simulink model "chalgyafzintegrationkrrhe"  (R2024b)
settings: Solver=ode4  StartTime=0.0  StopTime=150  FixedStep=0.001  RelTol=1e-3
values from neighbouring files (symbols this model uses):
  kappa = (dx .* d2y - dy .* d2x) ./          ((dx.^2 + dy.^2).^(3/2) + 1e-6)    [Buildmadrasspeedway.m]
  pathX = ppval(ppx,s)    [Buildmadrasspeedway.m]
  pathY = ppval(ppy,s)    [Buildmadrasspeedway.m]
  pathYaw = unwrap(atan2(dy,dx))    [Buildmadrasspeedway.m]
  s = 0:ds:t(end)    [Buildmadrasspeedway.m]
undefined symbols (not defined in the file or in its folder): v_ref
libraries: autolibsharedcoupling x1, vehdynlibsteering x1, autolibmappedmotor x1, vehdynlibdriver x1, autolibshared x1
(part 1 of 2)
settings Model: Creator=ASUS  LastModifiedBy=ASUS
settings DataIOCC: ReturnWorkspaceOutputs=off

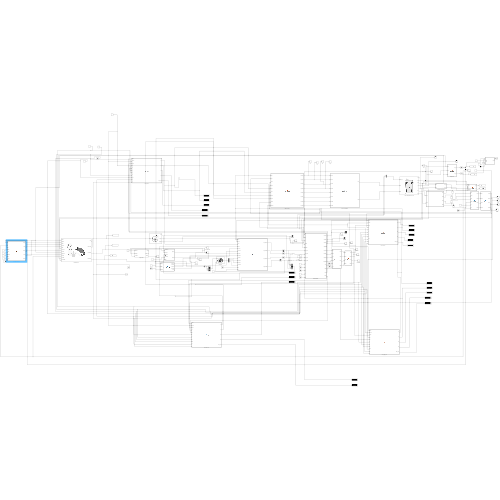
[thumbnail: Simulink's stored preview of the top-level diagram]
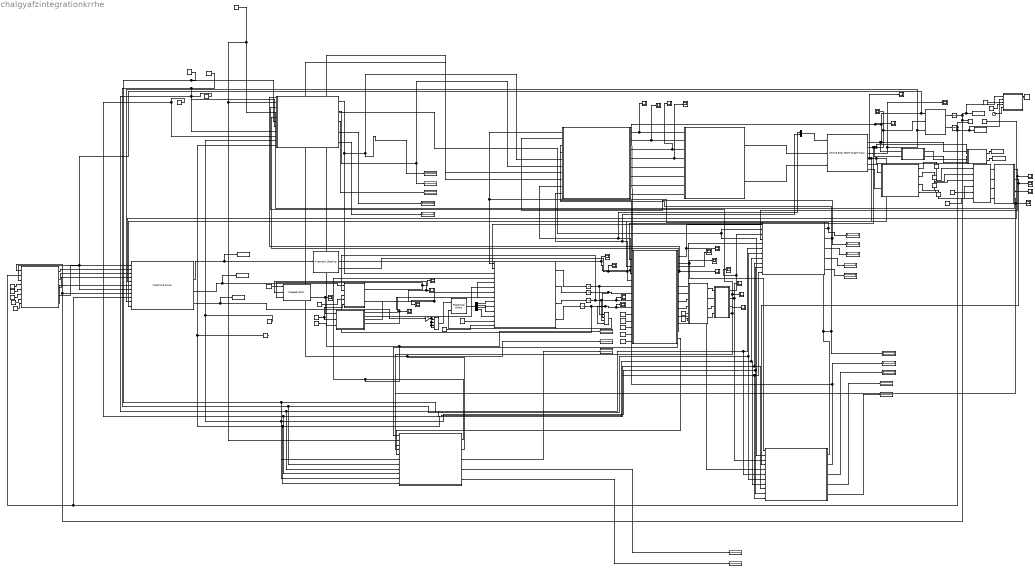
== system chalgyafzintegrationkrrhe ==
  Alpha RR : Scope
  Alpha Rl : Scope
  Bodytoworld : MATLAB Function  TreatAsAtomicUnit=on
  Clock : Clock
  Constant : Constant  Value=pathX(1)
  Constant1 : Constant  Value=0.10
  Constant10 : Constant  Value=0.001
  Constant11 : Constant  Value=0.08
  Constant12 : Constant  Value=0.03
  Constant13 : Constant  Value=0.001
  Constant14 : Constant  Value=kappa
  Constant15 : Constant  Value=pathX
  Constant16 : Constant  Value=0.3
  Constant17 : Constant  Value=0
  Constant18 : Constant  Value=pathY
  Constant19 : Constant  Value=pathYaw
  Constant2 : Constant  Value=0.08
  Constant20 : Constant  Value=v_ref
  Constant21 : Constant  Value=60
  Constant22 : Constant  Value=6
  Constant23 : Constant  Value=0.95
  Constant24 : Constant
  Constant25 : Constant  Value=pathY(1)
  Constant3 : Constant  Value=0.30
  Constant31 : Constant  Value=0.8
  Constant32 : Constant  Value=0.8
  Constant33 : Constant  Value=1.2
  Constant34 : Constant  Value=1.2
  Constant35 : Constant  Value=0.3
  Constant4 : Constant
  Constant5 : Constant  Value=1e7
  Constant6 : Constant  Value=200
  Constant7 : Constant  Value=0
  Constant9 : Constant
  Demux : Demux
  Disc Brake : autolibsharedcoupling/Rotational Brake  BrakeType=Disc  rotType=No inertia  extInfo=off  Iyy=1  br=1e-3  omegao=0  mu_static=0.4  mu_kinetic=0.35  disk_abore=0.02  Rm=0.08  num_pads=2  drum_abore=0.0508  drum_a=0.123  drum_c=0.212  drum_r=0.15  drum_theta1=0  drum_theta2=126  brake_p_bpt=[1 11.4736842105263 21.9473684210526 32.4210526315789 42.8947368421053 53.3684210526316 63.8421052631579 74.3157894736842 84.7894736842105 95.2631578947368 105.736842105263 116.210526315789 126.684210526316 137.157894736842 147.631578947368 158.105263157895 168.578947368421 179.052631578947 189.526315789474 200]  brake_n_bpt=[0 52.6315789473684 105.263157894737 157.894736842105 210.526315789474 263.157894736842 315.789473684211 368.421052631579 421.052631578947 473.684210526316 526.315789473684 578.947368421053 631.578947368421 684.210526315789 736.842105263158 789.473684210526 842.105263157895 894.736842105263 947.368421052632 1000]  f_brake_t=[43.4900602404453 42.5056030554862 41.5350898940194 40.5780454442085 39.6340111501808 38.7025443887544 37.7832176914519 36.8756180088306 35.9793460143796 35.0940154454303 34.2192524787115 33.3546951383474 32.4999927342521 31.6548053290159 30.8188032315107 29.991666515561 29.1730845621415 28.362755623661 27.5603864089927 26.765691687993;498.991217495636 487.695866636631 476.560505099801 465.579679307235 454.748127933653 444.060772460445 433.51270824929 423.099196101319 412.81565427025 402.657650900201 392.620896861006 382.701238955775 372.894653477208 363.197240090814 353.605216024701 344.114910546964 334.722759712992 325.425301366216 316.219170376863 307.10109410434;954.492374750826 932.886130217776 911.585920305583 890.581313170261 869.862244717126 849.419000532136 829.242198807128 809.322774193808 789.651962526121 770.221286354971 751.0225412433 732.047782773203 713.289314220164 694.739674852612 676.391628817892 658.238154578366 640.272434863842 622.48784710877 604.877954344734 587.436496520688;1409.99353200602 1378.07639379892 1346.61133551136 1315.58294703329 1284.9763615006 1254.77722860383 1224.97168936497 1195.5463522863 1166.48827078199 1137.78492180974 1109.42418562559 1081.39432659063 1053.68397496312 1026.28210961441 999.178041611083 972.361398609768 945.822110014692 919.550392851325 893.536738312604 867.771898937035;1865.49468926121 1823.26665738007 1781.63675071715 1740.58458089631 1700.09047828407 1660.13545667552 1620.7011799228 1581.76993037878 1543.32457903786 1505.34855726451 1467.82583000789 1430.74087040806 1394.07863570608 1357.82454437621 1321.96445440427 1286.48464264117 1251.37178516554 1216.61293859388 1182.19552228048 1148.10730135338;2320.9958465164 2268.45692096121 2216.66216592293 2165.58621475934 2115.20459506754 2065.49368474721 2016.43067048064 1967.99350847127 1920.16088729373 1872.91219271928 1826.22747439018 1780.08741422549 1734.47329644903 1689.36697913801 1644.75086719747 1600.60788667257 1556.92146031639 1513.67548433643 1470.85430624835 1428.44270376973;2776.49700377159 2713.64718454235 2651.68758112871 2590.58784862237 2530.31871185102 2470.8519128189 2412.16016103848 2354.21708656376 2296.9971955496 2240.47582817405 2184.62911877248 2129.43395804292 2074.86795719199 2020.9094138998 1967.53727999066 1914.73113070398 1862.47113546724 1810.73803007899 1759.51309021622 1708.77810618608;3231.99816102678 3158.8374481235 3086.71299633449 3015.58948248539 2945.43282863449 2876.21014089059 2807.88965159632 2740.44066465625 2673.83350380547 2608.03946362882 2543.03076315477 2478.78050186034 2415.26261793494 2352.4518486616 2290.32369278385 2228.85437473538 2168.02081061809 2107.80057582154 2048.17187418409 1989.11350860242;3687.49931828197 3604.02771170464 3521.73841154027 3440.59111634842 3360.54694541796 3281.56836896228 3203.61914215416 3126.66424274874 3050.66981206134 2975.60309908359 2901.43240753707 2828.12704567777 2755.6572786779 2683.9942834234 2613.11010557704 2542.97761876678 2473.57048576894 2404.8631215641 2336.83065815196 2269.44891101877;4143.00047553716 4049.21797528579 3956.76382674606 3865.59275021144 3775.66106220143 3686.92659703397 3599.34863271199 3512.88782084123 3427.50612031721 3343.16673453836 3259.83405191936 3177.4735894952 3096.05193942085 3015.5367181852 2935.89651837023 2857.10086279818 2779.12016091979 2701.92566730665 2625.48944211983 2549.78431343512;4598.50163279235 4494.40823886693 4391.78924195184 4290.59438407447 4190.77517898491 4092.28482510566 3995.07812326983 3899.11139893372 3804.34242857308 3710.73036999313 3618.23569630166 3526.82013331263 3436.44660016381 3347.079152947 3258.68293116342 3171.22410682959 3084.66983607064 2998.98821304921 2914.1482260877 2830.11971585147;5054.00279004754 4939.59850244808 4826.81465715762 4715.59601793749 4605.88929576838 4497.64305317735 4390.80761382767 4285.3349770262 4181.17873682896 4078.2940054479 3976.63734068395 3876.16667713006 3776.84126090677 3678.62158770879 3581.46934395661 3485.34735086099 ...(+2764 chars)]  aMode=2
      settings: LibrarySourceBlock=vehdynlibbrake/Disc Brake
  Display{,1..19} (20 alike) : Display
  FZFL : Scope
  FZFR : Scope
  FZRL : Scope
  FZRR : Scope
  "Force FWF and FWR " : MATLAB Function  TreatAsAtomicUnit=on
  Front_Left_tire : MATLAB Function  TreatAsAtomicUnit=on
  Front_Right_Tire : MATLAB Function  TreatAsAtomicUnit=on
  Gain : Gain  Gain=8e+6
  Integrator{,1..2,4} (4 alike) : Integrator  InitialCondition=0.1/0.3
  Integrator3 : Integrator  InitialCondition=pathX(1)
  Integrator5 : Integrator  InitialCondition=pathY(1)
  KAPPA FL : Scope
  KAPPA FR : Scope
  KAPPA RL : Scope
  KAPPA RR : Scope
  Kinematic Steering : vehdynlibsteering/Kinematic Steering  StrgType=Ackerman  StrgRatioType=Constant  Loc=Front  NrmlFctr=0.01  TrckWdth=1.2  WhlBase=1.6  Db=0  StrgRng=deg2rad(25)  StrgAngBpts="[-6.2832   -5.0265   -3.7699   -2.5133   -1.2566         0    1.2566    2.5133    3.7699    5.0265    6.2832]"  StrgRatioTbl=|  StrgRatio=1  PctAckIn=off  PctAck=100  PctAckTbl=ones(1,11)*100  StrgArmLngth=0.1  RckCsLngth=0.5  TieRodLngth=0.248  D=0.2  PnnRadius=0.00085818  PnnRadiusTbl="[0.0055    0.0055    0.0056    0.0057    0.0058    0.0057    0.0057    0.0057    0.0056    0.0055    0.0055]"  RodLngth=0.1  ParaArmLngth=0.9  aMode=2
      | [13.5000   13.3750   13.2500   13.1250   13.0000   13.0000   13.0000   13.1250   13.2500   13.3750   13.5000
      | ]
  MATLAB Function : MATLAB Function  TreatAsAtomicUnit=on
  MATLAB Function1 : MATLAB Function  TreatAsAtomicUnit=on
  MATLAB Function10 : MATLAB Function  TreatAsAtomicUnit=on
  MATLAB Function2 : MATLAB Function  TreatAsAtomicUnit=on
  MATLAB Function3 : MATLAB Function  TreatAsAtomicUnit=on  SystemSampleTime=0.001
  MATLAB Function4 : MATLAB Function  TreatAsAtomicUnit=on
  MATLAB Function5 : MATLAB Function  TreatAsAtomicUnit=on  SystemSampleTime=0.001
  MATLAB Function6 : MATLAB Function  TreatAsAtomicUnit=on
  MATLAB Function7 : MATLAB Function  TreatAsAtomicUnit=on
  MATLAB Function8 : MATLAB Function  TreatAsAtomicUnit=on
  MATLAB Function9 : MATLAB Function  TreatAsAtomicUnit=on
  Mapped Motor : autolibmappedmotor/Mapped Motor  w_Tmax_bp_ext=w_Tmax_bp  Tmax_w_V_ext=Tmax_w_V  w_Tmin_bp_ext=w_Tmin_bp  Tmin_w_V_ext=Tmin_w_V  port_config=Speed  param_by=Maximum torque and power  w_t=[ 0 375 750 800 ]  T_t=[0.09 0.08 0.07 0]  torque_max=60  power_max=35000  SpreadsheetTqLimitsFileName=MotorCalibrationImportData.xlsx  Tmax_w_V=[0.09 0.09 0.09;0.08 0.08 0.08;0.07 0.07 0.07;0 0 0]  w_Tmax_bp=[ 0 375 750 800 ]  V_Tmax_bp=[500 750 900]  Tmin_w_V=[-0.09 -0.09 -0.09;-0.08 -0.08 -0.08;-0.07 -0.07 -0.07;0 0 0]  w_Tmin_bp=[ 0 375 750 800 ]  V_Tmin_bp=[500 750 900]  Tc=0.02  param_loss=Single efficiency measurement  SpreadsheetLossFileName=MotorCalibrationImportData.xlsx  SpreadsheetEffFileName=MotorCalibrationImportData.xlsx  eff=100  w_eff=375  T_eff=0.08  Piron=0  Pbase=0  w_eff_bp=[-8000 -4000 0 4000 8000]  T_eff_bp=[0 0.03 0.06 0.09]  Temp_eff_bp=[233.15 293.15 373.15]  V_eff_bp=[500 700 900]  losses_table=[1.49 1.67 2.21 3.10; 0.42 0.69 1.14 2.03; 0.06 0.24 0.78 1.68; 0.42 0.69 1.14 2.03; 1.49 1.67 2.21 3.10]  losses_table_3d=cat(3,1.05*[1.49 1.67 2.21 3.10; 0.42 0.69 1.14 2.03; 0.06 0.24 0.78 1.68; 0.42 0.69 1.14 2.03; 1.49 1.67 2.21 3.10],[1.49 1.67 2.21 3.10; 0.42 0.69 1.14 2.03; 0.06 0.24 0.78 1.68; 0.42 0.69 1.14 2.03; 1.49 1.67 2.21 3.10],1.03*[1.49 1.67 2.21 3.10; 0.42 0.69 1.14 2.03; 0.06 0.24 0.78 1.68; 0.42 0.69 1.14 2.03; 1.49 1.67 2.21 3.10])  losses_table_4d=cat(4,cat(3,[1.5645 0.441 0.063 0.441 1.5645;1.7535 0.7245 0.252 0.7245 1.7535;2.3205 1.197 0.819 1.197 2.3205;3.255 2.1315 1.764 2.1315 3.255],[1.5645 0.441 0.063 0.441 1.5645;1.7535 0.7245 0.252 0.7245 1.7535;2.3205 1.197 0.819 1.197 2.3205;3.255 2.1315 1.764 2.1315 3.255],[1.5645 0.441 0.063 0.441 1.5645;1.7535 0.7245 0.252 0.7245 1.7535;2.3205 1.197 0.819 1.197 2.3205;3.255 2.1315 1.764 2.1315 3.255]),cat(3,[1.49 0.42 0.06 0.42 1.49;1.67 0.69 0.24 0.69 1.67;2.21 1.14 0.78 1.14 2.21;3.1 2.03 1.68 2.03 3.1],[1.49 0.42 0.06 0.42 1.49;1.67 0.69 0.24 0.69 1.67;2.21 1.14 0.78 1.14 2.21;3.1 2.03 1.68 2.03 3.1],[1.49 0.42 0.06 0.42 1.49;1.67 0.69 0.24 0.69 1.67;2.21 1.14 0.78 1.14 2.21;3.1 2.03 1.68 2.03 3.1]),cat(3,[1.5347 0.4326 0.0618 0.4326 1.5347;1.7201 0.7107 0.2472 0.7107 1.7201;2.2763 1.1742 0.8034 1.1742 2.2763;3.193 2.0909 1.7304 2.0909 3.193],[1.5347 0.4326 0.0618 0.4326 1.5347;1.7201 0.7107 0.2472 0.7107 1.7201;2.2763 1.1742 0.8034 1.1742 2.2763;3.193 2.0909 1.7304 2.0909 3.193],[1.5347 0.4326 0.0618 0.4326 1.5347;1.7201 0.7107 0.2472 0.7107 1.7201;2.2763 1.1742 0.8034 1.1742 2.2763;3.193 2.0909 1.7304 2.0909 3.193]))  efficiency_table=[95 95 95 95; 95 95 95 95; 95 95 95 95; 95 95 95 95; 95 95 95 95]  efficiency_table_3d=cat(3,90*ones(5,4),95*ones(5,4),92*ones(5,4))  efficiency_table_4d=cat(4,cat(3,90*ones(5,4)',90*ones(5,4)',90*ones(5,4)'),cat(3,95*ones(5,4)',95*ones(5,4)',95*ones(5,4)'),cat(3,92*ones(5,4)',92*ones(5,4)',92*ones(5,4)'))  J=5e-6  b=1e-5  omega_o=0  T_t_extended=[0 0.07 0.08 0.09 0.08 0.07 0]  w_t_extended=[-800 -750 -375 0 375 750 800]  KLossIron=0  KLossCopper=0  x_w_eff_vec=[-8000 -4000 0 4000 8000]  x_T_eff_vec=[-0.09 -0.06 -0.03 0 0.03 0.06 0.09]  x_tmp_eff_vec=[233.15 293.15 373.15]  x_V_eff_vec=[500 700 900]  x_losses_mat=[3.1 2.21 1.67 1.49 1.67 2.21 3.1;2.03 1.14 0.69 0.42 0.69 1.14 2.03;1.68 0.78 0.24 0.06 0.24 0.78 1.68;2.03 1.14 0.69 0.42 0.69 1.14 2.03;3.1 2.21 1.67 1.49 1.67 2.21 3.1]  x_losses_mat_3d=cat(3,[3.255 2.3205 1.7535 1.5645 1.7535 2.3205 3.255;2.1315 1.197 0.7245 0.441 0.7245 1.197 2.1315;1.764 0.819 0.252 0.063 0.252 0.819 1.764;2.1315 1.197 0.7245 0.441 0.7245 1.197 2.1315;3.255 2.3205 1.7535 1.5645 1.7535 2.3205 3.255],[3.1 2.21 1.67 1.49 1.67 2.21 3.1;2.03 1.14 0.69 0.42 0.69 1.14 2.03;1.68 0.78 0.24 0.06 0.24 0.78 1.68;2.03 1.14 0.69 0.42 0.69 1.14 2.03;3.1 2.21 1.67 1.49 1.67 2.21 3.1],[3.193 2.2763 1.7201 1.5347 1.7201 2.2763 3.193;2.0909 1.1742 0.7107 0.4326 0.7107 1.1742 2.0909;1.7304 0.8034 0.2472 0.0618 0.2472 0.8034 1.7304;2.0909 1.1742 0.7107 0.4326 0.7107 1.1742 2.0909;3.193 2.2763 1.7201 1.5347 1.7201 2.2763 3.193])  x_losses_mat_4d=cat(4,cat(3,[1.5645 0.441 0.063 0.441 1.5645;1.7535 0.7245 0.252 0.7245 1.7535;2.3205 1.197 0.819 1.197 2.3205;3.255 2.1315 1.764 2.1315 3.255],[1.5645 0.441 0.063 0.441 1.5645;1.7535 0.7245 0.252 0.7245 1.7535;2.3205 1.197 0.819 1.197 2.3205;3.255 2.1315 1.764 2.1315 3.255],[1.5645 0.441 0.063 0.441 1.5645;1.7535 0.7245 0.252 0.7245 1.7535;2.3205 1.197 0.819 1.197 2.3205;3.255 2.1315 1.764 2.1315 3.255]),cat(3,[1.49 0.42 0.06 0.42 1.49;1.67 0.69 0.24 0.69 1.67;2.21 1.14 0.78 1.14 2.21;3.1 2.03 1.68 2.03 3.1],[1.49 0.42 0.06 0.42 1.49;1.67 0.69 0.24 0.69 1.67;2.21 1.14 0.78 1.14 2.21;3.1 2.03 1.68 2.03 3.1],[1.49 0.42 0.06 0.42 1.49;1.67 0.69 0.24 0.69 1.67;2.21 1.14 0.78 1.14 2.21;3.1 2.03 1.68 2.03 3.1]),cat(3,[1.5347 0.4326 0.0618 0.4326 1.5347;1.7201 0.7107 0.2472 0.7107 1.7201;2.2763 1.1742 0.8034 1.1742 2.2763;3.193 2.0909 1.7304 2.0909 3.193],[1.5347 0.4326 0.0618 0.4326 1.5347;1.7201 0.7107 0.2472 0.7107 1.7201;2.2763 1.1742 0.8034 1.1742 2.2763;3.193 2.0909 1.7304 2.0909 3.193],[1.5347 0.4326 0.0618 0.4326 1.5347;1.7201 0.7107 0.2472 0.7107 1.7201;2.2763 1.1742 0.8034 1.1742 2.2763;3.193 2.0909 1.7304 2.0909 3.193]))  CalLossMapData={}  CalLossWithTempMapData={}  aMode=2  RefBlkName='autolibmappedmotor/Mapped Motor'
      settings: LibrarySourceBlock=vdynlib/Powertrain/Propulsion/Mapped Motor
  Memory{,1..3} (4 alike) : Memory  InitialCondition=735.38
  Motor torque : Scope
  Mtr speed : Scope
  Mux : Mux  Inputs=2
  Omega RL : Scope
  Omega RR : Scope
  PSI : Scope
  Predictive Driver : vehdynlibdriver/Predictive Driver  extAccelOvr=off  extDecelOvr=off  extAccelHld=off  extDecelHld=off  extAccelZero=off  extDecelZero=off  extSteerOvr=off  extSteerHld=off  extSteerZero=off  cntrlType=PI  cntrlTypeLat=Stanley  shftType=None  coordMode=SAE J670 (Z-down)  refType=Reference pose  velUnits=m/s  angUnits=rad  gearOut=off  steerOut=off  Kp=10  Ki=5  Kff=.1  Kg=0  VehVelVec=[0 100]  KffVec=[.1 .1]  KpVec=[10 10]  KiVec=[5 5]  KgVec=[0 0]  vnom=25  Kaw=1  tauerr=.01  tau=0.1  L=3  Kpt=3000  aR=200  bR=2.5  cR=.5  g=9.81  vecPose=off  dynamMode=on  PositionGainF=2.5  PositionGainR=2.5  YawRateGain=.2  DelayGain=.2  enableDrift=off  BetaRef=20*pi/180  KpBeta=1  KpDrift=2  KdDrift=1  KpPsi=6  KOmega=30  tOmega=1  a=0.8  b=0.8  m=300  Cy_f=45456  Cy_r=70933  I=4013  Ksteer=18  theta=45*pi/180  Idl=3  Re=.3  lambda_mu=1  GearInit=0  tShift=.1  pdlVec=[0.1 0.4 0.5 0.9]  upShftTbl=[-1 12.9375 26.4375 39.9375 51.18749999999999 62.4375 72.84375 83.25;-1 16.3125 29.8125 43.3125 54.5624 65.8125 76.78125 87.75;-1 19.6875 33.1875 46.68749999999999 57.9375 69.1875 80.71875 92.25;-1 33 52.5 77.25 100.5 138.75 161.875 185]  dwnShftTbl=[-1 12.9375 26.4375 39.9375 51.18749999999999 62.4375 72.84375 83.25;-1 16.3125 29.8125 43.3125 54.5624 65.8125 76.78125 87.75;-1 19.6875 33.1875 46.68749999999999 57.9375 69.1875 80.71875 92.25;-1 33 52.5 77.25 100.5 138.75 161.875 185]  tClutch=.5  tRev=.5  tPark=120  UpGearVec="[0  1  2  3  4  5  6  7]"  DownGearVec="[1  2  3  4  5  6  7  8]"  aMode=2
  "Rear_left tire " : MATLAB Function  TreatAsAtomicUnit=on
  Rear_right_tire : MATLAB Function  TreatAsAtomicUnit=on
  Stop Simulation : Stop
  Tdrive RL : Scope
  Tdrive RR : Scope
  To Workspace : ToWorkspace  VariableName=X_sim  SampleTime=-1
      settings: Decimation=10
  To Workspace1 : ToWorkspace  VariableName=Y_sim  SampleTime=-1
      settings: Decimation=10
  To Workspace2 : ToWorkspace  VariableName=X_sim1  SampleTime=-1
      settings: Decimation=10
  To Workspace3 : ToWorkspace  VariableName=Y_sim1  SampleTime=-1
      settings: Decimation=10
  To Workspace5 : ToWorkspace  VariableName=Steer  SampleTime=-1
      settings: Decimation=10
  To Workspace6 : ToWorkspace  VariableName=Accel  SampleTime=-1
      settings: Decimation=10
  To Workspace7 : ToWorkspace  VariableName=Decel  SampleTime=-1
      settings: Decimation=10
  Trq commmand : Scope
  Vector Concatenate : Concatenate  NumInputs=4
  Vector Concatenate1 : Concatenate  NumInputs=4
  Vehicle Body 3DOF Dual Track : autolibshared/Vehicle Body 3DOF Single Track  trackMode=Dual  inputMode=External forces  frontSteerMode=on  rearSteerMode=off  windMode=off  muMode=off  extFMode=off  extMMode=off  htchFMode=off  htchMMode=off  extXo=off  extpsio=off  extxdoto=off  extro=off  extYo=off  extTamb=off  extydoto=off  aMode=2  NF=2  NR=2  m=300  a=0.8  b=0.8  h=0.3  dh=1  hh=0.2  X_o=pathX(1)  xdot_o=0.1  CalphaMode=off  sigmaMode=on  d=0  hl=0  w=[1.2,1.2]  Cy_f=12e3  Cy_r=11e3  sigma_f=.1  sigma_r=.1  alpha_f_brk=[-.1 .1]  Cy_f_data=[-9e3 9e3]  alpha_r_brk=[-.1 .1]  Cy_r_data=[-9e3 9e3]  Y_o=pathY(1)  ydot_o=0  Izz=120  psi_o=pathYaw(1)  r_o=0  Af=0  Cd=0  Cl=0  Cpm=0  beta_w=[0 0.01:0.01:0.3]  Cs=[0:0.03:0.9]  Cym=[0 1e-6:0.01:0.3]  Pabs=101325  Tair=273  g=9.81  mu=1  xdot_tol=.01  Fznom=5000  Fxtire_sat=7e4  Fytire_sat=7e4  longOff=0  latOff=0  vertOff=0  wrapAng=off
      settings: LibrarySourceBlock=vehdynlibeom/Vehicle Body 3DOF Dual Track
  VehicleVelocityDerivative : MATLAB Function  TreatAsAtomicUnit=on
  Wheel kinematics : MATLAB Function  TreatAsAtomicUnit=on
  XY Graph : Record  FileSettingsInternal="{\"entries\":[{\"content\":{\"excelSettings\":{\"content\":{},\"type\":\"Streamout.ExcelSettings\"}},\"type\":\"Streamout.FileSettingStorage\",\"uuid\":\"\"}],\"packageUris\":[\"http:\\/\\/schema.mathworks.com\\/mf0\\/streamout_blocks\\/R2020a\"],\"version\":\"1.0\"}"  Layout=[1 1]  SignalsInternal="{\"entries\":[{\"content\":{\"signals\":[{\"content\":{\"blockPath\":[],\"dimensions\":[1],\"domain\":\"\",\"lineColor\":\"#a2142f\",\"plots\":[ 1 ],\"port\":1,\"sid\":[\"\"],\"signalID\":1,\"signalName\":\"X_sim\"},\"type\":\"RecordBlkView.Signal\",\"uuid\":\"\"},{\"content\":{\"blockPath\":[],\"dimensions\":[1],\"domain\":\"\",\"lineColor\":\"#139fff\",\"plots\":[ 1 ],\"port\":2,\"sid\":[\"\"],\"signalID\":2,\"signalName\":\"Y_sim\"},\"type\":\"RecordBlkView.Signal\",\"uuid\":\"\"}]},\"type\":\"RecordBlkView.InputSignals\",\"uuid\":\"\"}],\"packageUris\":[\"http:\\/\\/schema.mathworks.com\\/mf0\\/streamout_blocks\\/R2020a\"],\"version\":\"1.0\"}"  VisualizationBindings="{\"xyplotplugin\":{\"info\":[{\"series\":[{\"bindingParametersList\":[{\"parameter\":\"X-Axis\",\"signalID\":1,\"signalName\":\"X_sim\"},{\"parameter\":\"Y-Axis\",\"signalID\":2,\"signalName\":\"Y_sim\"}],\"seriesID\":0}],\"subplotID\":1}]}}"  CompatibilityTag=XY
  Xdot2 : Scope
  alpahFL : Scope
  alpha FR : Scope
  fx fl : Scope
  fxfr : Scope
  fyfl : Scope
  fyfr : Scope
  "left angle " : Scope
  r : Scope
  "right angle " : Scope
  "wheel to vehicle " : MATLAB Function  TreatAsAtomicUnit=on
  ydot : Scope
  wires:
  Mux/1 -> Vehicle Body 3DOF Dual Track/1
  Integrator4/1 -> Vector Concatenate/4, Omega RR/1, Wheel kinematics/9(omegaRR), MATLAB Function6/3(omegaRR)
  MATLAB Function4/1(kFLs) -> KAPPA FL/1, Front_Left_tire/3(kappa)
  "Force FWF and FWR "/2(FwR) -> Vehicle Body 3DOF Dual Track/3
  Vehicle Body 3DOF Dual Track/7 -> MATLAB Function/2(FzR)
  Integrator2/1 -> Omega RL/1, Wheel kinematics/8(omegaRL), Vector Concatenate/3, MATLAB Function6/2(omegaRL)
  MATLAB Function4/2(kFRs) -> KAPPA FR/1, Front_Right_Tire/3(kappa)
  MATLAB Function4/3(kRLs) -> KAPPA RL/1, "Rear_left tire "/3(kappa)
  MATLAB Function4/4(kRRs) -> Rear_right_tire/3(kappa), KAPPA RR/1
  Integrator/1 -> Vector Concatenate/1, Wheel kinematics/6(omegaFL)
  Vehicle Body 3DOF Dual Track/4 -> Predictive Driver/10, Bodytoworld/3(psi), PSI/1
  Vehicle Body 3DOF Dual Track/3 -> VehicleVelocityDerivative/2(Uy), MATLAB Function10/2(ydot), Bodytoworld/2(ydot), ydot/1, Wheel kinematics/2(Uy)
  Vehicle Body 3DOF Dual Track/2 -> VehicleVelocityDerivative/1(Ux), MATLAB Function10/1(xdot), Predictive Driver/7, MATLAB Function8/3(Vx), Bodytoworld/1(xdot), Wheel kinematics/1(Ux), Xdot2/1
  Vehicle Body 3DOF Dual Track/5 -> r/1, Predictive Driver/11, MATLAB Function10/3(r), Wheel kinematics/3(r)
  Vehicle Body 3DOF Dual Track/6 -> MATLAB Function/1(FzF)
  Kinematic Steering/3 -> "right angle "/1, Wheel kinematics/5(deltaFR), Mux/2, "wheel to vehicle "/10(deltaFR)
  Front_Left_tire/2(Fy) -> Display16/1, "wheel to vehicle "/2(FyFL)
  "wheel to vehicle "/4(FyVehFR) -> fyfr/1, "Force FWF and FWR "/4(FyVehFR)
  Constant6/1 -> "Rear_left tire "/11(n), Front_Right_Tire/11(n), Front_Left_tire/11(n), Rear_right_tire/11(n)
  Rear_right_tire/5(slide_count) -> Display9/1
  Rear_right_tire/2(Fy) -> Display6/1, "wheel to vehicle "/8(FyRR)
  Constant16/1 -> MATLAB Function1/13(Rw)
  Wheel kinematics/12(VcRR) -> Rear_right_tire/5(Vc)
  Constant34/1 -> Wheel kinematics/13(tr)
  Integrator1/1 -> Vector Concatenate/2, Wheel kinematics/7(omegaFR)
  "Rear_left tire "/3(Mz) -> Display2/1
  Constant5/1 -> Front_Left_tire/10(cp), Front_Right_Tire/10(cp), Rear_right_tire/10(cp), "Rear_left tire "/10(cp)
  MATLAB Function1/2(omegaDotFR) -> Integrator1/1
  Front_Right_Tire/2(Fy) -> Display11/1, "wheel to vehicle "/4(FyFR)
  Front_Right_Tire/3(Mz) -> Display12/1
  "Rear_left tire "/1(Fx) -> MATLAB Function1/3(FxRL), "wheel to vehicle "/5(FxRL), Display/1
  Constant35/1 -> Wheel kinematics/14(Rw)
  Constant32/1 -> Wheel kinematics/11(lr)
  MATLAB Function1/4(omegaDotRR) -> Integrator4/1
  Front_Right_Tire/1(Fx) -> MATLAB Function1/2(FxFR), Display10/1, "wheel to vehicle "/3(FxFR)
  Constant3/1 -> "Rear_left tire "/8(re), Front_Left_tire/8(re), Front_Right_Tire/8(re), Rear_right_tire/8(re)
  "Rear_left tire "/5(slide_count) -> Display4/1
  "wheel to vehicle "/6(FyVehRL) -> "Force FWF and FWR "/6(FyVehRL)
  Wheel kinematics/9(VcFL) -> Front_Left_tire/5(Vc)
  Constant4/1 -> "Rear_left tire "/9(mu0), Front_Left_tire/9(mu0), Front_Right_Tire/9(mu0), Rear_right_tire/9(mu0)
  Constant7/1 -> Front_Right_Tire/2(gamma), Front_Left_tire/2(gamma), Rear_right_tire/2(gamma), "Rear_left tire "/2(gamma)
  "wheel to vehicle "/1(FxVehFL) -> fx fl/1, "Force FWF and FWR "/1(FxVehFL)
  "wheel to vehicle "/3(FxVehFR) -> fxfr/1, "Force FWF and FWR "/3(FxVehFR)
  Rear_right_tire/3(Mz) -> Display7/1
  Front_Left_tire/1(Fx) -> Display15/1, MATLAB Function1/1(FxFL), "wheel to vehicle "/1(FxFL)
  MATLAB Function1/1(omegaDotFL) -> Integrator/1
  Wheel kinematics/3(alphaRL) -> Alpha Rl/1, "Rear_left tire "/1(alpha)
  Rear_right_tire/1(Fx) -> MATLAB Function1/4(FxRR), Display5/1, "wheel to vehicle "/7(FxRR)
  Front_Left_tire/3(Mz) -> Display17/1
  Constant1/1 -> "Rear_left tire "/6(a), Front_Left_tire/6(a), Front_Right_Tire/6(a), Rear_right_tire/6(a)
  Wheel kinematics/11(VcRL) -> "Rear_left tire "/5(Vc)
  Front_Left_tire/5(slide_count) -> Display19/1
  Kinematic Steering/2 -> "left angle "/1, Wheel kinematics/4(deltaFL), Mux/1, "wheel to vehicle "/9(deltaFL)
  Constant31/1 -> Wheel kinematics/10(lf)
  MATLAB Function1/3(omegaDotRL) -> Integrator2/1
  Wheel kinematics/4(alphaRR) -> Alpha RR/1, Rear_right_tire/1(alpha)
  "wheel to vehicle "/5(FxVehRL) -> "Force FWF and FWR "/5(FxVehRL)
  Front_Right_Tire/4(Mx) -> Display13/1
  Wheel kinematics/1(alphaFL) -> alpahFL/1, Front_Left_tire/1(alpha)
  Front_Right_Tire/5(slide_count) -> Display14/1
  Rear_right_tire/4(Mx) -> Display8/1
  "Rear_left tire "/4(Mx) -> Display3/1
  Constant2/1 -> "Rear_left tire "/7(b), Front_Left_tire/7(b), Front_Right_Tire/7(b), Rear_right_tire/7(b)
  Wheel kinematics/10(VcFR) -> Front_Right_Tire/5(Vc)
  "wheel to vehicle "/8(FyVehRR) -> "Force FWF and FWR "/8(FyVehRR)
  Constant33/1 -> Wheel kinematics/12(tf)
  Constant9/1 -> MATLAB Function1/14(Iw)
  "wheel to vehicle "/7(FxVehRR) -> "Force FWF and FWR "/7(FxVehRR)
  "wheel to vehicle "/2(FyVehFL) -> fyfl/1, "Force FWF and FWR "/2(FyVehFL)
  Wheel kinematics/2(alphaFR) -> alpha FR/1, Front_Right_Tire/1(alpha)
  "Rear_left tire "/2(Fy) -> "wheel to vehicle "/6(FyRL), Display1/1
  Front_Left_tire/4(Mx) -> Display18/1
  "Force FWF and FWR "/1(FwF) -> Vehicle Body 3DOF Dual Track/2
  MATLAB Function/4(FzRR) -> Memory3/1
  MATLAB Function/1(FzFL) -> Memory/1
  MATLAB Function/2(FzFR) -> Memory2/1
  MATLAB Function/3(FzRL) -> Memory1/1
  Memory/1 -> MATLAB Function2/1(FzFL)
  Memory1/1 -> MATLAB Function2/3(FzRL)
  Memory2/1 -> MATLAB Function2/2(FzFR)
  Memory3/1 -> MATLAB Function2/4(FzRR)
  MATLAB Function3/3(FzRLs) -> "Rear_left tire "/4(Fz), FZRL/1
  MATLAB Function3/1(FzFLs) -> FZFL/1, Front_Left_tire/4(Fz)
  MATLAB Function3/2(FzFRs) -> FZFR/1, Front_Right_Tire/4(Fz)
  MATLAB Function3/4(FzRRs) -> Rear_right_tire/4(Fz), FZRR/1
  Constant10/1 -> MATLAB Function2/5(dt)
  Constant11/1 -> MATLAB Function2/6(tau)
  MATLAB Function2/1(FzFLf) -> MATLAB Function3/1(FzFL)
  MATLAB Function2/2(FzFRf) -> MATLAB Function3/2(FzFR)
  MATLAB Function2/3(FzRLf) -> MATLAB Function3/3(FzRL)
  MATLAB Function2/4(FzRRf) -> MATLAB Function3/4(FzRR)
  Wheel kinematics/8(kappaRR) -> MATLAB Function5/4(kRR)
  Wheel kinematics/7(kappaRL) -> MATLAB Function5/3(kRL)
  Wheel kinematics/6(kappaFR) -> MATLAB Function5/2(kFR)
  Wheel kinematics/5(kappaFL) -> MATLAB Function5/1(kFL)
  Disc Brake/1 -> Demux/1
  MATLAB Function5/1(kFLf) -> MATLAB Function4/1(kFL)
  MATLAB Function5/2(kFRf) -> MATLAB Function4/2(kFR)
  MATLAB Function5/3(kRLf) -> MATLAB Function4/3(kRL)
  MATLAB Function5/4(kRRf) -> MATLAB Function4/4(kRR)
  Constant12/1 -> MATLAB Function5/6(tau)
  Constant13/1 -> MATLAB Function5/5(dt)
  Mapped Motor/3 -> MATLAB Function7/1(MtrTrq), Motor torque/1
  Constant21/1 -> MATLAB Function6/4(TmotorMax)
  Constant22/1 -> MATLAB Function7/2(Ndiff), MATLAB Function6/5(Ndiff)
  Constant23/1 -> MATLAB Function7/3(etaDiff)
  MATLAB Function6/1(TrqCmd) -> Mapped Motor/3, Trq commmand/1
  MATLAB Function6/2(MtrSpd) -> Mtr speed/1, Mapped Motor/2
  Constant24/1 -> Mapped Motor/1
  MATLAB Function7/1(TdriveFL) -> MATLAB Function1/5(TdriveFL)
  MATLAB Function7/2(TdriveFR) -> MATLAB Function1/6(TdriveFR)
  MATLAB Function7/3(TdriveRL) -> MATLAB Function1/7(TdriveRL), Tdrive RL/1
  MATLAB Function7/4(TdriveRR) -> MATLAB Function1/8(TdriveRR), Tdrive RR/1
  Predictive Driver/3 -> To Workspace6/1, MATLAB Function6/1(throttleCmd)
  Vector Concatenate/1 -> Disc Brake/2
  Predictive Driver/4 -> To Workspace7/1, Gain/1
  Gain/1 -> Vector Concatenate1/4, Vector Concatenate1/3, Vector Concatenate1/2, Vector Concatenate1/1
  Vector Concatenate1/1 -> Disc Brake/1
  Demux/1 -> MATLAB Function1/9(TbrakeFL)
  Demux/2 -> MATLAB Function1/10(TbrakeFR)
  Demux/3 -> MATLAB Function1/11(TbrakeRL)
  Demux/4 -> MATLAB Function1/12(TbrakeRR)
  Bodytoworld/1(Xdot_w) -> Integrator3/1
  Bodytoworld/2(Ydot_w) -> Integrator5/1
  Integrator3/1 -> XY Graph/1, MATLAB Function8/1(X), Predictive Driver/8, MATLAB Function9/1(X), To Workspace/1  "X_sim"
  Integrator5/1 -> MATLAB Function9/2(Y), To Workspace1/1, Predictive Driver/9, MATLAB Function8/2(Y), XY Graph/2  "Y_sim"
  Constant17/1 -> Predictive Driver/5
  Predictive Driver/2 -> To Workspace5/1, Kinematic Steering/1
  Constant15/1 -> MATLAB Function8/4(pathX)
  Constant18/1 -> MATLAB Function8/5(pathY)
  Constant19/1 -> MATLAB Function8/6(pathYaw)
  Constant20/1 -> MATLAB Function8/7(v_ref)
  MATLAB Function8/1(LongRef) -> Predictive Driver/2
  MATLAB Function8/2(LatRef) -> Predictive Driver/3
  MATLAB Function8/3(YawRef) -> Predictive Driver/4
  MATLAB Function8/4(VelRef) -> Predictive Driver/1
  Constant14/1 -> MATLAB Function8/8(kappa)
  MATLAB Function8/5(CurvRef) -> Predictive Driver/6
  Constant/1 -> MATLAB Function9/3(pathX1)
  Constant25/1 -> MATLAB Function9/4(pathY1)
  Clock/1 -> MATLAB Function9/5(t)
  MATLAB Function9/1(stop) -> Stop Simulation/1
  VehicleVelocityDerivative/1(Ux_dot) -> MATLAB Function10/4(xdot_deriv)
  VehicleVelocityDerivative/2(Uy_dot) -> MATLAB Function10/5(ydot_deriv)
  MATLAB Function10/2(ay_G) -> To Workspace3/1
  MATLAB Function10/1(ax_G) -> To Workspace2/1

== matlab function chalgyafzintegrationkrrhe/Rear_right_tire ==
  data: alpha input; Fx output; gamma input; kappa input; Fz input; Vc input; a input; b input; re input; mu0 input; cp input; n input; Fy output; Mz output; Mx output; slide_count output
function [Fx,Fy,Mz,Mx,slide_count] = tread_model( ...
                alpha,...
                gamma,...
                kappa,...
                Fz,...
                Vc,...
                a,b,re,...
                mu0,...
                cp,...
                n)

%%%%%%%%%%%%%%%%%%%%%%%%%%%%%%%%%%%%%%%%%%%%%%%%%%%%%%%%%%%%
% CONTACT PATCH
%%%%%%%%%%%%%%%%%%%%%%%%%%%%%%%%%%%%%%%%%%%%%%%%%%%%%%%%%%%%

xb = linspace(a,-a,n);

dx = abs(xb(2)-xb(1));

%%%%%%%%%%%%%%%%%%%%%%%%%%%%%%%%%%%%%%%%%%%%%%%%%%%%%%%%%%%%
% ROLLING KINEMATICS
%%%%%%%%%%%%%%%%%%%%%%%%%%%%%%%%%%%%%%%%%%%%%%%%%%%%%%%%%%%%

Vr = Vc/(1-kappa);

Omega = Vr/re;

dt = dx/Vr;

%%%%%%%%%%%%%%%%%%%%%%%%%%%%%%%%%%%%%%%%%%%%%%%%%%%%%%%%%%%%
% SLIP VELOCITIES
%%%%%%%%%%%%%%%%%%%%%%%%%%%%%%%%%%%%%%%%%%%%%%%%%%%%%%%%%%%%

Vsx = -Vc*kappa;

Vsy = -Vc*tan(alpha);

%%%%%%%%%%%%%%%%%%%%%%%%%%%%%%%%%%%%%%%%%%%%%%%%%%%%%%%%%%%%
% MULTI ROW TREAD
%%%%%%%%%%%%%%%%%%%%%%%%%%%%%%%%%%%%%%%%%%%%%%%%%%%%%%%%%%%%

nRows = 11;

yrow = linspace(-b,b,nRows);

dyrow = (2*b)/(nRows-1);

%%%%%%%%%%%%%%%%%%%%%%%%%%%%%%%%%%%%%%%%%%%%%%%%%%%%%%%%%%%%
% OUTPUT INITIALIZATION
%%%%%%%%%%%%%%%%%%%%%%%%%%%%%%%%%%%%%%%%%%%%%%%%%%%%%%%%%%%%

Fx = 0;
Fy = 0;
Mz = 0;
Mx = 0;

slide_count = 0;

%%%%%%%%%%%%%%%%%%%%%%%%%%%%%%%%%%%%%%%%%%%%%%%%%%%%%%%%%%%%
% PRESSURE NORMALIZATION
%%%%%%%%%%%%%%%%%%%%%%%%%%%%%%%%%%%%%%%%%%%%%%%%%%%%%%%%%%%%

ShapeSum = 0;

for r = 1:nRows

    yb0 = yrow(r);

    for i = 1:n

        px = max(0,1-(xb(i)/a)^2);

        py = sqrt(max(0,1-(yb0/b)^2));

        ShapeSum = ShapeSum + px*py*dx*dyrow;

    end
end

qz0 = Fz/ShapeSum;

%%%%%%%%%%%%%%%%%%%%%%%%%%%%%%%%%%%%%%%%%%%%%%%%%%%%%%%%%%%%
% MAIN LOOP
%%%%%%%%%%%%%%%%%%%%%%%%%%%%%%%%%%%%%%%%%%%%%%%%%%%%%%%%%%%%

for r = 1:nRows

    yb0 = yrow(r);

    ex = 0;
    ey = 0;

    for i = 1:n

        px = max(0,1-(xb(i)/a)^2);

        py = sqrt(max(0,1-(yb0/b)^2));

        qz = qz0*px*py;

        if qz <= 0
            continue
        end

        dybdx = (xb(i)/re)*sin(gamma);

        Vbx = Vsx + yb0*Omega*sin(gamma);

        Vby = Vsy - Vr*dybdx;

        %%%%%%%%%%%%%%%%%%%%%%%%%%%%%%%%%%%%%%%%%%%%%%%%%%%%
        % CONSTANT FRICTION
        %%%%%%%%%%%%%%%%%%%%%%%%%%%%%%%%%%%%%%%%%%%%%%%%%%%%

        qlimit = mu0*qz;

        Dsx = Vbx*dt;

        Dsy = Vby*dt;

        ex_trial = ex - Dsx;

        ey_trial = ey - Dsy;

        qx_trial = cp*ex_trial;

        qy_trial = cp*ey_trial;

        qtrial = hypot(qx_trial,qy_trial);

        %%%%%%%%%%%%%%%%%%%%%%%%%%%%%%%%%%%%%%%%%%%%%%%%%%%%
        % ADHESION
        %%%%%%%%%%%%%%%%%%%%%%%%%%%%%%%%%%%%%%%%%%%%%%%%%%%%

        if qtrial <= qlimit

            ex = ex_trial;
            ey = ey_trial;

            qx = cp*ex;
            qy = cp*ey;

        %%%%%%%%%%%%%%%%%%%%%%%%%%%%%%%%%%%%%%%%%%%%%%%%%%%%
        % SLIDING
        %%%%%%%%%%%%%%%%%%%%%%%%%%%%%%%%%%%%%%%%%%%%%%%%%%%%

        else

            slide_count = slide_count + 1;

            e_i = qlimit/cp;

            norm_trial = hypot(ex_trial,ey_trial);

            if norm_trial > 1e-12

                ex = e_i*ex_trial/norm_trial;

                ey = e_i*ey_trial/norm_trial;

            else

                ex = 0;
                ey = 0;

            end

            qx = cp*ex;
            qy = cp*ey;

        end

        dA = dx*dyrow;

        dFx = qx*dA;
        dFy = qy*dA;

        Fx = Fx + dFx;
        Fy = Fy + dFy;

        Mz = Mz + xb(i)*dFy - yb0*dFx;

        Mx = Mx + yb0*dFy;

    end
end

end

== matlab function chalgyafzintegrationkrrhe/Front_Right_Tire ==
  data: alpha input; Fx output; gamma input; kappa input; Fz input; Vc input; a input; b input; re input; mu0 input; cp input; n input; Fy output; Mz output; Mx output; slide_count output
function [Fx,Fy,Mz,Mx,slide_count] = tread_model( ...
                alpha,...
                gamma,...
                kappa,...
                Fz,...
                Vc,...
                a,b,re,...
                mu0,...
                cp,...
                n)

%%%%%%%%%%%%%%%%%%%%%%%%%%%%%%%%%%%%%%%%%%%%%%%%%%%%%%%%%%%%
% CONTACT PATCH
%%%%%%%%%%%%%%%%%%%%%%%%%%%%%%%%%%%%%%%%%%%%%%%%%%%%%%%%%%%%

xb = linspace(a,-a,n);

dx = abs(xb(2)-xb(1));

%%%%%%%%%%%%%%%%%%%%%%%%%%%%%%%%%%%%%%%%%%%%%%%%%%%%%%%%%%%%
% ROLLING KINEMATICS
%%%%%%%%%%%%%%%%%%%%%%%%%%%%%%%%%%%%%%%%%%%%%%%%%%%%%%%%%%%%

Vr = Vc/(1-kappa);

Omega = Vr/re;

dt = dx/Vr;

%%%%%%%%%%%%%%%%%%%%%%%%%%%%%%%%%%%%%%%%%%%%%%%%%%%%%%%%%%%%
% SLIP VELOCITIES
%%%%%%%%%%%%%%%%%%%%%%%%%%%%%%%%%%%%%%%%%%%%%%%%%%%%%%%%%%%%

Vsx = -Vc*kappa;

Vsy = -Vc*tan(alpha);

%%%%%%%%%%%%%%%%%%%%%%%%%%%%%%%%%%%%%%%%%%%%%%%%%%%%%%%%%%%%
% MULTI ROW TREAD
%%%%%%%%%%%%%%%%%%%%%%%%%%%%%%%%%%%%%%%%%%%%%%%%%%%%%%%%%%%%

nRows = 11;

yrow = linspace(-b,b,nRows);

dyrow = (2*b)/(nRows-1);

%%%%%%%%%%%%%%%%%%%%%%%%%%%%%%%%%%%%%%%%%%%%%%%%%%%%%%%%%%%%
% OUTPUT INITIALIZATION
%%%%%%%%%%%%%%%%%%%%%%%%%%%%%%%%%%%%%%%%%%%%%%%%%%%%%%%%%%%%

Fx = 0;
Fy = 0;
Mz = 0;
Mx = 0;

slide_count = 0;

%%%%%%%%%%%%%%%%%%%%%%%%%%%%%%%%%%%%%%%%%%%%%%%%%%%%%%%%%%%%
% PRESSURE NORMALIZATION
%%%%%%%%%%%%%%%%%%%%%%%%%%%%%%%%%%%%%%%%%%%%%%%%%%%%%%%%%%%%

ShapeSum = 0;

for r = 1:nRows

    yb0 = yrow(r);

    for i = 1:n

        px = max(0,1-(xb(i)/a)^2);

        py = sqrt(max(0,1-(yb0/b)^2));

        ShapeSum = ShapeSum + px*py*dx*dyrow;

    end
end

qz0 = Fz/ShapeSum;

%%%%%%%%%%%%%%%%%%%%%%%%%%%%%%%%%%%%%%%%%%%%%%%%%%%%%%%%%%%%
% MAIN LOOP
%%%%%%%%%%%%%%%%%%%%%%%%%%%%%%%%%%%%%%%%%%%%%%%%%%%%%%%%%%%%

for r = 1:nRows

    yb0 = yrow(r);

    ex = 0;
    ey = 0;

    for i = 1:n

        px = max(0,1-(xb(i)/a)^2);

        py = sqrt(max(0,1-(yb0/b)^2));

        qz = qz0*px*py;

        if qz <= 0
            continue
        end

        dybdx = (xb(i)/re)*sin(gamma);

        Vbx = Vsx + yb0*Omega*sin(gamma);

        Vby = Vsy - Vr*dybdx;

        %%%%%%%%%%%%%%%%%%%%%%%%%%%%%%%%%%%%%%%%%%%%%%%%%%%%
        % CONSTANT FRICTION
        %%%%%%%%%%%%%%%%%%%%%%%%%%%%%%%%%%%%%%%%%%%%%%%%%%%%

        qlimit = mu0*qz;

        Dsx = Vbx*dt;

        Dsy = Vby*dt;

        ex_trial = ex - Dsx;

        ey_trial = ey - Dsy;

        qx_trial = cp*ex_trial;

        qy_trial = cp*ey_trial;

        qtrial = hypot(qx_trial,qy_trial);

        %%%%%%%%%%%%%%%%%%%%%%%%%%%%%%%%%%%%%%%%%%%%%%%%%%%%
        % ADHESION
        %%%%%%%%%%%%%%%%%%%%%%%%%%%%%%%%%%%%%%%%%%%%%%%%%%%%

        if qtrial <= qlimit

            ex = ex_trial;
            ey = ey_trial;

            qx = cp*ex;
            qy = cp*ey;

        %%%%%%%%%%%%%%%%%%%%%%%%%%%%%%%%%%%%%%%%%%%%%%%%%%%%
        % SLIDING
        %%%%%%%%%%%%%%%%%%%%%%%%%%%%%%%%%%%%%%%%%%%%%%%%%%%%

        else

            slide_count = slide_count + 1;

            e_i = qlimit/cp;

            norm_trial = hypot(ex_trial,ey_trial);

            if norm_trial > 1e-12

                ex = e_i*ex_trial/norm_trial;

                ey = e_i*ey_trial/norm_trial;

            else

                ex = 0;
                ey = 0;

            end

            qx = cp*ex;
            qy = cp*ey;

        end

        dA = dx*dyrow;

        dFx = qx*dA;
        dFy = qy*dA;

        Fx = Fx + dFx;
        Fy = Fy + dFy;

        Mz = Mz + xb(i)*dFy - yb0*dFx;

        Mx = Mx + yb0*dFy;

    end
end

end

== matlab function chalgyafzintegrationkrrhe/wheel to vehicle  ==
  data: FxFL input; FxVehFL output; FyFL input; FxFR input; FyFR input; FxRL input; FyRL input; FxRR input; FyRR input; deltaFL input; deltaFR input; FyVehFL output; FxVehFR output; FyVehFR output; FxVehRL output; FyVehRL output; FxVehRR output; FyVehRR output
function [FxVehFL,FyVehFL,FxVehFR,FyVehFR, ...
          FxVehRL,FyVehRL,FxVehRR,FyVehRR] = TransformForces( ...
          FxFL,FyFL,FxFR,FyFR, ...
          FxRL,FyRL,FxRR,FyRR, ...
          deltaFL,deltaFR)
%#codegen

% Front-left wheel frame to vehicle frame
FxVehFL = FxFL*cos(deltaFL) - FyFL*sin(deltaFL);
FyVehFL = -FxFL*sin(deltaFL) + FyFL*cos(deltaFL);

% Front-right wheel frame to vehicle frame
FxVehFR = FxFR*cos(deltaFR) - FyFR*sin(deltaFR);
FyVehFR = -FxFR*sin(deltaFR) + FyFR*cos(deltaFR);

% Rear wheels are not steered
FxVehRL = FxRL;
FyVehRL = FyRL;

FxVehRR = FxRR;
FyVehRR = FyRR;

end

== matlab function chalgyafzintegrationkrrhe/Force FWF and FWR  ==
  data: FxVehFL input; FwF output; FyVehFL input; FxVehFR input; FyVehFR input; FxVehRL input; FyVehRL input; FxVehRR input; FyVehRR input; FwR output
function [FwF,FwR] = BuildForceInputs( ...
    FxVehFL,FyVehFL,FxVehFR,FyVehFR, ...
    FxVehRL,FyVehRL,FxVehRR,FyVehRR)
%#codegen

% Correct Vehicle Body 3DOF format:
% Row 1 = left wheel
% Row 2 = right wheel
% Column 1 = Fx
% Column 2 = Fy

FwF = [FxVehFL  FyVehFL;
       FxVehFR  FyVehFR];

FwR = [FxVehRL  FyVehRL;
       FxVehRR  FyVehRR];

end

== matlab function chalgyafzintegrationkrrhe/MATLAB Function ==
  data: FzF input; FzFL output; FzR input; FzFR output; FzRL output; FzRR output
function [FzFL,FzFR,FzRL,FzRR] = SplitFz(FzF,FzR)
%#codegen

FzFL = 0.0;
FzFR = 0.0;
FzRL = 0.0;
FzRR = 0.0;

% Linear indexing works for both row and column vectors
FzFL = FzF(1);
FzFR = FzF(2);

FzRL = FzR(1);
FzRR = FzR(2);

end

== matlab function chalgyafzintegrationkrrhe/MATLAB Function1 ==
  data: FxFL input; omegaDotFL output; FxFR input; FxRL input; FxRR input; TdriveFL input; TdriveFR input; TdriveRL input; TdriveRR input; TbrakeFL input; TbrakeFR input; TbrakeRL input; TbrakeRR input; Rw input; Iw input; omegaDotFR output; omegaDotRL output; omegaDotRR output
function [omegaDotFL,omegaDotFR,omegaDotRL,omegaDotRR] = WheelDynamics( ...
    FxFL,FxFR,FxRL,FxRR, ...
    TdriveFL,TdriveFR,TdriveRL,TdriveRR, ...
    TbrakeFL,TbrakeFR,TbrakeRL,TbrakeRR, ...
    Rw,Iw)

omegaDotFL = 0.0;
omegaDotFR = 0.0;
omegaDotRL = 0.0;
omegaDotRR = 0.0;

omegaDotFL = (TdriveFL - TbrakeFL - FxFL*Rw)/Iw;
omegaDotFR = (TdriveFR - TbrakeFR - FxFR*Rw)/Iw;
omegaDotRL = (TdriveRL - TbrakeRL - FxRL*Rw)/Iw;
omegaDotRR = (TdriveRR - TbrakeRR - FxRR*Rw)/Iw;

end

== matlab function chalgyafzintegrationkrrhe/MATLAB Function2 ==
  data: FzFL input; FzFLf output; FzFR input; FzRL input; FzRR input; dt input; tau input; FzFRf output; FzRLf output; FzRRf output
function [FzFLf,FzFRf,FzRLf,FzRRf] = FzLowPass( ...
    FzFL,FzFR,FzRL,FzRR,dt,tau)
%#codegen

persistent zFL zFR zRL zRR initialized

if isempty(initialized)
    zFL = FzFL;
    zFR = FzFR;
    zRL = FzRL;
    zRR = FzRR;
    initialized = true;
end

alpha = dt/(tau + dt);

zFL = zFL + alpha*(FzFL - zFL);
zFR = zFR + alpha*(FzFR - zFR);
zRL = zRL + alpha*(FzRL - zRL);
zRR = zRR + alpha*(FzRR - zRR);

FzFLf = zFL;
FzFRf = zFR;
FzRLf = zRL;
FzRRf = zRR;

end

== matlab function chalgyafzintegrationkrrhe/MATLAB Function3 ==
  data: FzFL input; FzFLs output; FzFR input; FzRL input; FzRR input; FzFRs output; FzRLs output; FzRRs output
function [FzFLs,FzFRs,FzRLs,FzRRs] = FzSafety(FzFL,FzFR,FzRL,FzRR)
%#codegen

FzMin = 50.0;

FzFLs = max(FzFL,FzMin);
FzFRs = max(FzFR,FzMin);
FzRLs = max(FzRL,FzMin);
FzRRs = max(FzRR,FzMin);

end

== matlab function chalgyafzintegrationkrrhe/MATLAB Function4 ==
  data: kFL input; kFLs output; kFR input; kRL input; kRR input; kFRs output; kRLs output; kRRs output
function [kFLs,kFRs,kRLs,kRRs] = KappaSafety(kFL,kFR,kRL,kRR)
%#codegen

kMin = -0.30;
kMax =  0.30;

kFLs = min(max(kFL,kMin),kMax);
kFRs = min(max(kFR,kMin),kMax);
kRLs = min(max(kRL,kMin),kMax);
kRRs = min(max(kRR,kMin),kMax);

end

== matlab function chalgyafzintegrationkrrhe/MATLAB Function5 ==
  data: kFL input; kFLf output; kFR input; kRL input; kRR input; dt input; tau input; kFRf output; kRLf output; kRRf output
function [kFLf,kFRf,kRLf,kRRf] = KappaLowPass(kFL,kFR,kRL,kRR,dt,tau)
%#codegen

persistent zFL zFR zRL zRR initialized

if isempty(initialized)
    zFL = kFL;
    zFR = kFR;
    zRL = kRL;
    zRR = kRR;
    initialized = true;
end

alpha = dt/(tau + dt);

zFL = zFL + alpha*(kFL - zFL);
zFR = zFR + alpha*(kFR - zFR);
zRL = zRL + alpha*(kRL - zRL);
zRR = zRR + alpha*(kRR - zRR);

kFLf = zFL;
kFRf = zFR;
kRLf = zRL;
kRRf = zRR;

end

== matlab function chalgyafzintegrationkrrhe/MATLAB Function6 ==
  data: throttleCmd input; TrqCmd output; omegaRL input; omegaRR input; TmotorMax input; Ndiff input; MtrSpd output
function [TrqCmd, MtrSpd] = EV_Command_And_Speed( ...
    throttleCmd, omegaRL, omegaRR, TmotorMax, Ndiff)
%#codegen

%% Safe inputs
throttle = min(max(throttleCmd, 0.0), 1.0);
Tmax     = max(TmotorMax, 0.0);
N        = max(Ndiff, 0.01);

%% Throttle to motor torque request
TrqCmd = throttle*Tmax;

%% Open-differential speed relationship
omegaCarrier = 0.5*(omegaRL + omegaRR);
MtrSpd       = N*omegaCarrier;

end

== matlab function chalgyafzintegrationkrrhe/MATLAB Function7 ==
  data: MtrTrq input; TdriveFL output; Ndiff input; etaDiff input; TdriveFR output; TdriveRL output; TdriveRR output; Taxle output
function [TdriveFL, TdriveFR, TdriveRL, TdriveRR, Taxle] = ...
    Open_Differential_Torque(MtrTrq, Ndiff, etaDiff)
%#codegen

%% Safe parameters
N   = max(Ndiff, 0.01);
eta = min(max(etaDiff, 0.0), 1.0);

%% Total torque after reduction
Taxle = MtrTrq*N*eta;

%% Rear-wheel-drive configuration
TdriveFL = 0.0;
TdriveFR = 0.0;

%% Ideal open differential: equal wheel torque
TdriveRL = 0.5*Taxle;
TdriveRR = 0.5*Taxle;

end

== matlab function chalgyafzintegrationkrrhe/Bodytoworld ==
  data: xdot input; Xdot_w output; ydot input; psi input; Ydot_w output
function [Xdot_w, Ydot_w] = BodyToWorld(xdot, ydot, psi)

Xdot_w = xdot*cos(psi) - ydot*sin(psi);
Ydot_w = xdot*sin(psi) + ydot*cos(psi);
